simulink model "observer"  (R2021a)
settings: Solver=VariableStepAuto  StartTime=0.0  StopTime=0.25  MaxStep=0.0001  RelTol=1e-3
values from neighbouring files (symbols this model uses):
  A = adj    [ceren_function.m]    (also in deneme.m = [-resi/L -1/L; 1/C 0]; get_mass_spring_model.m = [0 1 0 0; (-k1-k2)/m1 0 k2/m1 0; 0 0 0 1; k2/m2 0 -k2/m2 0]; matlab.mat = [0  -100; 1000  0])
  B = [1/L; 0]    [deneme.m]    (also in get_mass_spring_model.m = [0; 1/m1; 0; 0]; matlab.mat = [100 0])
  c = 200    [init_graph.m]    (also in matlab.mat = 10)
  C = [0 1]    [deneme.m]    (also in get_mass_spring_model.m = [1 0 0 0; 0 0 1 0]; matlab.mat)
  c_switch = 1    [matlab.mat]
  D = [0]    [deneme.m]    (also in get_mass_spring_model.m = [0; 0; 0;0]; matlab.mat = 0)
  F = F'    [init_graph.m]    (also in matlab.mat = [-0.0499875062461 -10.4868971814])
  K = [7.50549770549 2.31662479036]    [matlab.mat]
settings Model: Creator=umut  LastModifiedBy=umut

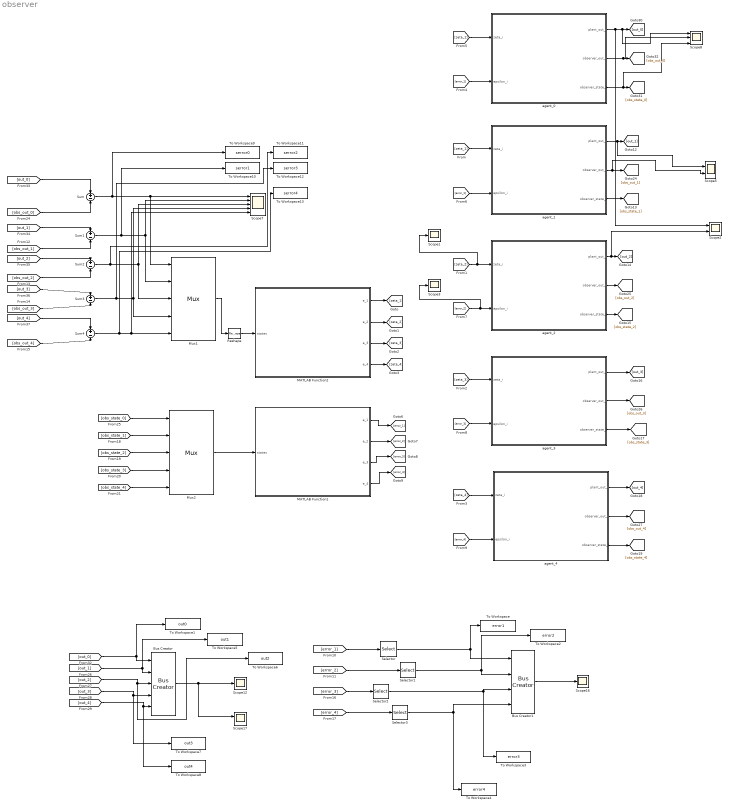
== system observer ==
  Bus Creator : BusCreator  Inputs=5
  Bus Creator1 : BusCreator  Inputs=4
  MATLAB Function1 : MATLAB Function  TreatAsAtomicUnit=on
  MATLAB Function2 : MATLAB Function  TreatAsAtomicUnit=on
  Mux1 : Mux  Inputs=5
  Mux2 : Mux  Inputs=5
  Reshape : Reshape  OutputDimensionality=Customize  OutputDimensions=[5,1]
  Scope{1,3,12,16} (4 alike) : Scope
  Scope17 : Scope  NumInputPorts=2
  Scope2 : Scope  NumInputPorts=2
  Scope5 : Scope  NumInputPorts=2
  Scope7 : Scope  NumInputPorts=5
  Scope8 : Scope  NumInputPorts=6
  Selector{,1..3} (4 alike) : Selector  InputPortWidth=2  IndexOptions=Starting index (dialog)  Indices=2  OutputSizes=1
  Sum{,1..4} (5 alike) : Sum  Inputs=+|-
  To Workspace : ToWorkspace  VariableName=error1  SampleTime=-1
      settings: Save2DSignal=2-D array (concatenate along first dimension)
  To Workspace1 : ToWorkspace  VariableName=out0  SampleTime=-1
      settings: Save2DSignal=2-D array (concatenate along first dimension)
  To Workspace10 : ToWorkspace  VariableName=serror1  SampleTime=-1
      settings: Save2DSignal=2-D array (concatenate along first dimension)
  To Workspace11 : ToWorkspace  VariableName=serror2  SampleTime=-1
      settings: Save2DSignal=2-D array (concatenate along first dimension)
  To Workspace12 : ToWorkspace  VariableName=serror3  SampleTime=-1
      settings: Save2DSignal=2-D array (concatenate along first dimension)
  To Workspace13 : ToWorkspace  VariableName=serror4  SampleTime=-1
      settings: Save2DSignal=2-D array (concatenate along first dimension)
  To Workspace2 : ToWorkspace  VariableName=error2  SampleTime=-1
      settings: Save2DSignal=2-D array (concatenate along first dimension)
  To Workspace3 : ToWorkspace  VariableName=error3  SampleTime=-1
      settings: Save2DSignal=2-D array (concatenate along first dimension)
  To Workspace4 : ToWorkspace  VariableName=error4  SampleTime=-1
      settings: Save2DSignal=2-D array (concatenate along first dimension)
  To Workspace5 : ToWorkspace  VariableName=out1  SampleTime=-1
      settings: Save2DSignal=2-D array (concatenate along first dimension)
  To Workspace6 : ToWorkspace  VariableName=out2  SampleTime=-1
      settings: Save2DSignal=2-D array (concatenate along first dimension)
  To Workspace7 : ToWorkspace  VariableName=out3  SampleTime=-1
      settings: Save2DSignal=2-D array (concatenate along first dimension)
  To Workspace8 : ToWorkspace  VariableName=out4  SampleTime=-1
      settings: Save2DSignal=2-D array (concatenate along first dimension)
  To Workspace9 : ToWorkspace  VariableName=serror0  SampleTime=-1
      settings: Save2DSignal=2-D array (concatenate along first dimension)
  agent_0 : Subsystem
  agent_1 : Subsystem
  agent_2 : Subsystem
  agent_3 : Subsystem
  agent_4 : Subsystem
  wires:
  MATLAB Function1/3(e_3) -> [error_3]
  MATLAB Function1/2(e_2) -> [error_2]
  MATLAB Function1/1(e_1) -> [error_1]
  MATLAB Function1/4(e_4) -> [error_4]
  [zeta_3] -> agent_3/1(zeta_i)
  [zeta_2] -> Scope1/1, agent_2/1(zeta_i)
  [zeta_4] -> agent_4/1(zeta_i)
  [error_3] -> agent_3/2(epsilon_i)
  [error_4] -> agent_4/2(epsilon_i)
  [error_2] -> Scope3/1, agent_2/2(epsilon_i)
  agent_1/3(observer_state_i) -> [obs_state_1]
  agent_2/1(plant_out_i) -> Scope2/2, [out_2]
  agent_2/3(observer_state_i) -> [obs_state_2]
  agent_3/1(plant_out_i) -> [out_3]
  agent_3/3(observer_state_i) -> [obs_state_3]
  agent_4/1(plant_out_i) -> [out_4]
  agent_4/3(observer_state_i) -> [obs_state_4]
  Mux1/1 -> Reshape/1
  Sum1/1 -> To Workspace10/1, Mux1/2, Scope7/2
  Sum2/1 -> To Workspace11/1, Scope7/3, Mux1/3
  Sum3/1 -> To Workspace12/1, Scope7/4, Mux1/4
  Sum4/1 -> To Workspace13/1, Scope7/5, Mux1/5
  agent_1/2(observer_out_i) -> Scope5/2, [obs_out_1]
  agent_2/2(observer_out_i) -> [obs_out_2]
  agent_3/2(observer_out_i) -> [obs_out_3]
  agent_4/2(observer_out_i) -> [obs_out_4]
  [obs_state_4] -> Mux2/5
  [obs_state_2] -> Mux2/3
  [obs_state_3] -> Mux2/4
  [obs_state_1] -> Mux2/2
  Mux2/1 -> MATLAB Function1/1(states)
  [error_1] -> agent_1/2(epsilon_i)
  [zeta_1] -> agent_1/1(zeta_i)
  agent_0/2(observer_out_i) -> Scope8/3, [obs_out_0]
  agent_0/3(observer_state_i) -> Scope8/6, [obs_state_0]
  Sum/1 -> To Workspace9/1, Mux1/1, Scope7/1
  [obs_state_0] -> Mux2/1
  [zeta_1] -> agent_0/1(zeta_i)
  [error_1] -> agent_0/2(epsilon_i)
  agent_0/1(plant_out_i) -> Scope2/1, Scope8/1, [out_0]
  [obs_out_0] -> Sum/2
  [out_0] -> Sum/1
  [obs_out_1] -> Sum1/2
  [out_1] -> Sum1/1
  [obs_out_2] -> Sum2/2
  [out_2] -> Sum2/1
  [obs_out_3] -> Sum3/2
  [out_3] -> Sum3/1
  [out_4] -> Sum4/1
  [obs_out_4] -> Sum4/2
  Reshape/1 -> MATLAB Function2/1(states)
  agent_1/1(plant_out_i) -> Scope5/1, [out_1]
  MATLAB Function2/3(e_3) -> [zeta_3]
  MATLAB Function2/4(e_4) -> [zeta_4]
  MATLAB Function2/2(e_2) -> [zeta_2]
  MATLAB Function2/1(e_1) -> [zeta_1]
  [out_3] -> To Workspace7/1, Bus Creator/4
  [out_4] -> To Workspace8/1, Bus Creator/5
  [out_2] -> To Workspace6/1, Bus Creator/3
  Bus Creator/1 -> Scope12/1, Scope17/1
  [out_0] -> Bus Creator/1, To Workspace1/1
  [out_1] -> Bus Creator/2, To Workspace5/1
  Selector/1 -> Bus Creator1/1, To Workspace/1
  Bus Creator1/1 -> Scope16/1
  Selector1/1 -> Bus Creator1/2, To Workspace2/1
  [error_1] -> Selector/1
  [error_2] -> Selector1/1
  [error_3] -> Selector2/1
  [error_4] -> Selector3/1
  Selector2/1 -> Bus Creator1/3, To Workspace3/1
  Selector3/1 -> To Workspace4/1, Bus Creator1/4

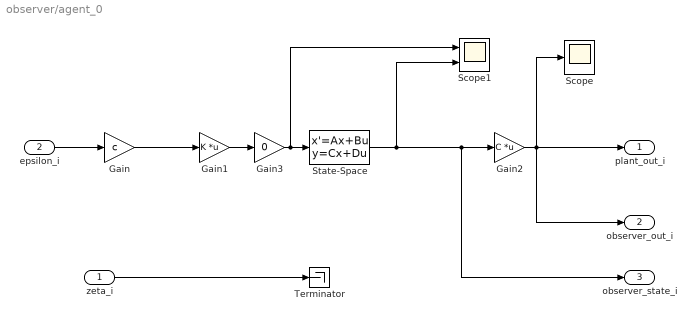
== system observer/agent_0 ==
  zeta_i : Inport
  epsilon_i : Inport  Port=2
  Gain : Gain  Gain=c
  Gain1 : Gain  Gain=K  Multiplication=Matrix(K*u)
  Gain2 : Gain  Gain=C  Multiplication=Matrix(K*u)
  Gain3 : Gain  Gain=0
  Scope : Scope
  Scope1 : Scope  NumInputPorts=2
  State-Space : StateSpace  A=A  B=B  C=eye(2)  D=[D;D]  InitialCondition=[20;0]
  Terminator : Terminator
  plant_out_i : Outport
  observer_out_i : Outport  Port=2
  observer_state_i : Outport  Port=3
  wires:
  epsilon_i/1 -> Gain/1
  zeta_i/1 -> Terminator/1
  State-Space/1 -> Scope1/2, Gain2/1, observer_state_i/1
  Gain/1 -> Gain1/1
  Gain2/1 -> Scope/1, plant_out_i/1, observer_out_i/1
  Gain1/1 -> Gain3/1
  Gain3/1 -> Scope1/1, State-Space/1

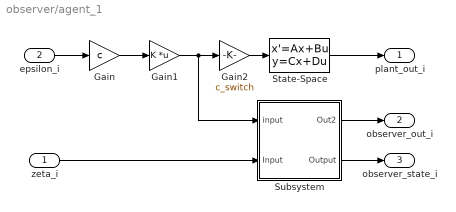
== system observer/agent_1 ==
  zeta_i : Inport
  epsilon_i : Inport  Port=2
  Gain : Gain  Gain=c
  Gain1 : Gain  Gain=K  Multiplication=Matrix(K*u)
  Gain2 : Gain  Gain=c_switch
  State-Space : StateSpace  A=A  B=B  C=C  D=D  InitialCondition=[30;80]
  Subsystem : Subsystem
  plant_out_i : Outport
  observer_out_i : Outport  Port=2
  observer_state_i : Outport  Port=3
  wires:
  epsilon_i/1 -> Gain/1
  State-Space/1 -> plant_out_i/1
  Subsystem/1(Out2) -> observer_out_i/1
  Subsystem/2(Output) -> observer_state_i/1
  zeta_i/1 -> Subsystem/2(Input)
  Gain/1 -> Gain1/1
  Gain1/1 -> Gain2/1, Subsystem/1(input)
  Gain2/1 -> State-Space/1

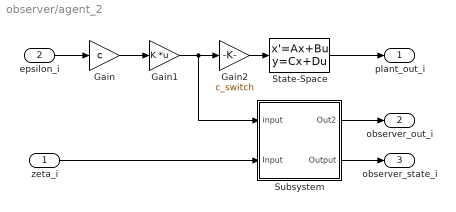
== system observer/agent_2 ==
  zeta_i : Inport
  epsilon_i : Inport  Port=2
  Gain : Gain  Gain=c
  Gain1 : Gain  Gain=K  Multiplication=Matrix(K*u)
  Gain2 : Gain  Gain=c_switch
  State-Space : StateSpace  A=A  B=B  C=C  D=D  InitialCondition=[30;100]
  Subsystem : Subsystem
  plant_out_i : Outport
  observer_out_i : Outport  Port=2
  observer_state_i : Outport  Port=3
  wires:
  epsilon_i/1 -> Gain/1
  State-Space/1 -> plant_out_i/1
  Subsystem/1(Out2) -> observer_out_i/1
  Subsystem/2(Output) -> observer_state_i/1
  zeta_i/1 -> Subsystem/2(Input)
  Gain/1 -> Gain1/1
  Gain1/1 -> Gain2/1, Subsystem/1(input)
  Gain2/1 -> State-Space/1

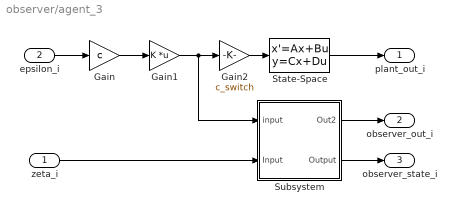
== system observer/agent_3 ==
  zeta_i : Inport
  epsilon_i : Inport  Port=2
  Gain : Gain  Gain=c
  Gain1 : Gain  Gain=K  Multiplication=Matrix(K*u)
  Gain2 : Gain  Gain=c_switch
  State-Space : StateSpace  A=A  B=B  C=C  D=D  InitialCondition=[20;60]
  Subsystem : Subsystem
  plant_out_i : Outport
  observer_out_i : Outport  Port=2
  observer_state_i : Outport  Port=3
  wires:
  epsilon_i/1 -> Gain/1
  State-Space/1 -> plant_out_i/1
  Subsystem/1(Out2) -> observer_out_i/1
  Subsystem/2(Output) -> observer_state_i/1
  zeta_i/1 -> Subsystem/2(Input)
  Gain/1 -> Gain1/1
  Gain1/1 -> Gain2/1, Subsystem/1(input)
  Gain2/1 -> State-Space/1

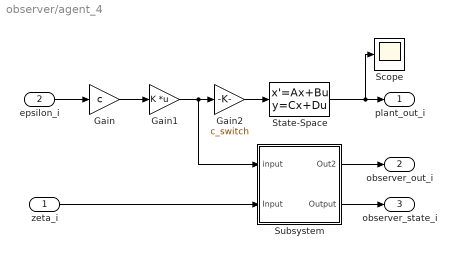
== system observer/agent_4 ==
  zeta_i : Inport
  epsilon_i : Inport  Port=2
  Gain : Gain  Gain=c
  Gain1 : Gain  Gain=K  Multiplication=Matrix(K*u)
  Gain2 : Gain  Gain=c_switch
  Scope : Scope
  State-Space : StateSpace  A=A  B=B  C=C  D=D  InitialCondition=[20;40]
  Subsystem : Subsystem
  plant_out_i : Outport
  observer_out_i : Outport  Port=2
  observer_state_i : Outport  Port=3
  wires:
  epsilon_i/1 -> Gain/1
  State-Space/1 -> Scope/1, plant_out_i/1
  Subsystem/1(Out2) -> observer_out_i/1
  Subsystem/2(Output) -> observer_state_i/1
  zeta_i/1 -> Subsystem/2(Input)
  Gain/1 -> Gain1/1
  Gain1/1 -> Gain2/1, Subsystem/1(input)
  Gain2/1 -> State-Space/1

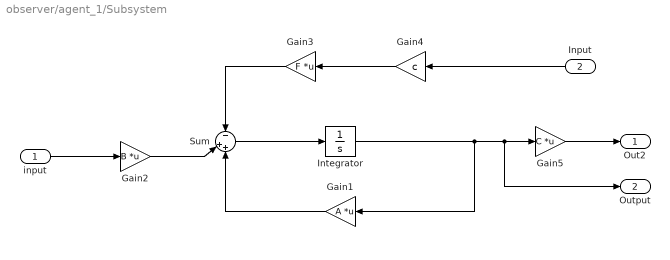
== system observer/agent_1/Subsystem ==
  input : Inport
  Input : Inport  Port=2
  Gain1 : Gain  Gain=A  Multiplication=Matrix(K*u)
  Gain2 : Gain  Gain=B  Multiplication=Matrix(K*u)
  Gain3 : Gain  Gain=F  Multiplication=Matrix(K*u)
  Gain4 : Gain  Gain=c
  Gain5 : Gain  Gain=C  Multiplication=Matrix(K*u)
  Integrator : Integrator
  Sum : Sum  Inputs=-|++
  Out2 : Outport
  Output : Outport  Port=2
  wires:
  Gain3/1 -> Sum/1
  Gain2/1 -> Sum/2
  input/1 -> Gain2/1
  Gain1/1 -> Sum/3
  Sum/1 -> Integrator/1
  Gain5/1 -> Out2/1
  Input/1 -> Gain4/1
  Gain4/1 -> Gain3/1
  Integrator/1 -> Output/1, Gain5/1, Gain1/1

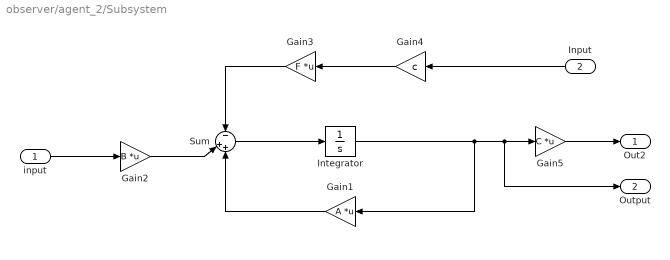
== system observer/agent_2/Subsystem ==
  input : Inport
  Input : Inport  Port=2
  Gain1 : Gain  Gain=A  Multiplication=Matrix(K*u)
  Gain2 : Gain  Gain=B  Multiplication=Matrix(K*u)
  Gain3 : Gain  Gain=F  Multiplication=Matrix(K*u)
  Gain4 : Gain  Gain=c
  Gain5 : Gain  Gain=C  Multiplication=Matrix(K*u)
  Integrator : Integrator
  Sum : Sum  Inputs=-|++
  Out2 : Outport
  Output : Outport  Port=2
  wires:
  Gain3/1 -> Sum/1
  Gain2/1 -> Sum/2
  input/1 -> Gain2/1
  Gain1/1 -> Sum/3
  Sum/1 -> Integrator/1
  Gain5/1 -> Out2/1
  Input/1 -> Gain4/1
  Gain4/1 -> Gain3/1
  Integrator/1 -> Output/1, Gain5/1, Gain1/1

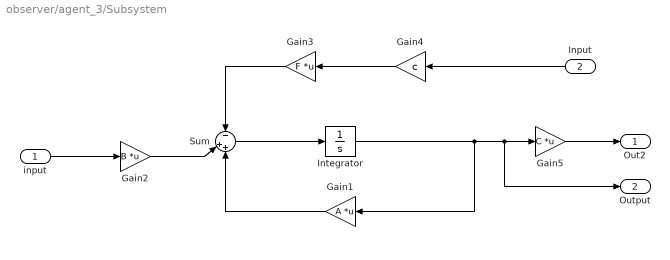
== system observer/agent_3/Subsystem ==
  input : Inport
  Input : Inport  Port=2
  Gain1 : Gain  Gain=A  Multiplication=Matrix(K*u)
  Gain2 : Gain  Gain=B  Multiplication=Matrix(K*u)
  Gain3 : Gain  Gain=F  Multiplication=Matrix(K*u)
  Gain4 : Gain  Gain=c
  Gain5 : Gain  Gain=C  Multiplication=Matrix(K*u)
  Integrator : Integrator
  Sum : Sum  Inputs=-|++
  Out2 : Outport
  Output : Outport  Port=2
  wires:
  Gain3/1 -> Sum/1
  Gain2/1 -> Sum/2
  input/1 -> Gain2/1
  Gain1/1 -> Sum/3
  Sum/1 -> Integrator/1
  Gain5/1 -> Out2/1
  Input/1 -> Gain4/1
  Gain4/1 -> Gain3/1
  Integrator/1 -> Output/1, Gain5/1, Gain1/1

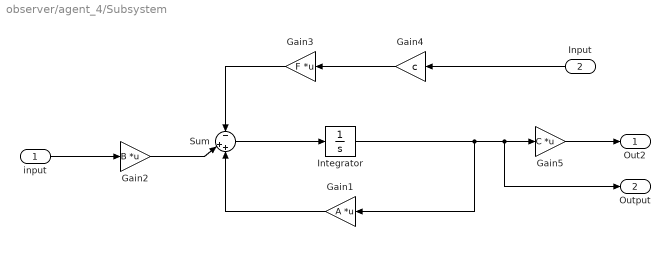
== system observer/agent_4/Subsystem ==
  input : Inport
  Input : Inport  Port=2
  Gain1 : Gain  Gain=A  Multiplication=Matrix(K*u)
  Gain2 : Gain  Gain=B  Multiplication=Matrix(K*u)
  Gain3 : Gain  Gain=F  Multiplication=Matrix(K*u)
  Gain4 : Gain  Gain=c
  Gain5 : Gain  Gain=C  Multiplication=Matrix(K*u)
  Integrator : Integrator
  Sum : Sum  Inputs=-|++
  Out2 : Outport
  Output : Outport  Port=2
  wires:
  Gain3/1 -> Sum/1
  Gain2/1 -> Sum/2
  input/1 -> Gain2/1
  Gain1/1 -> Sum/3
  Sum/1 -> Integrator/1
  Gain5/1 -> Out2/1
  Input/1 -> Gain4/1
  Gain4/1 -> Gain3/1
  Integrator/1 -> Output/1, Gain5/1, Gain1/1

== matlab function observer/MATLAB Function1 ==
  data: states input; e_1 output size=[2 1]; e_2 output size=[2 1]; e_3 output size=[2 1]; e_4 output size=[2 1]
function [e_1, e_2, e_3, e_4]  = calculate_neighborhood_error(states)
    adj = [ 0	1	1	1
            0   0   1   0
            1   0   0   0
            1   1   1   0]';
    
    pinnings = [1; 0; 0; 0];

    A = adj;
    G = pinnings;
    
    size_agents = 4;
    size_states = 2;
    
    error = zeros(size_states, size_agents);
    
    
    for i = 1 : size_agents
        error_temp = [0;0];
        for j = 1 : size_agents
            error_temp = error_temp + A(i, j) * (states((j)*2+1 : 2*(j+1)) - states((i)*2+1 : 2*(i+1)));
        end
        error_temp = error_temp + pinnings(i) * (states(1 : 2) - states((i)*2+1 : 2*(i+1)));
        error(:,i) = error_temp;
    end
    
    e_1 = error(:,1);
    e_2 = error(:,2);
    e_3 = error(:,3);
    e_4 = error(:,4);

end

== matlab function observer/MATLAB Function2 ==
  data: states input size=[5,1]; e_1 output size=[1, 1]; e_2 output size=[1, 1]; e_3 output size=[1, 1]; e_4 output size=[1, 1]
function [e_1, e_2, e_3, e_4]  = calculate_output_error(states)
    adj = [ 0	0	0	0
            1   0   0   0
            0   1   0   0
            0   0   1   0];
    
    pinnings = [1; 0; 0; 0];

    A = adj;
    G = pinnings;
    
    size_agents = 4;
    size_states = 1;
    
    error = zeros(size_states, size_agents);
    
    
    
    for i = 1 : size_agents
        error_temp = zeros(1,1);
        for j = 1 : size_agents
            term1 = (states(j+1) - states(i+1));
            error_temp = error_temp + A(i, j) * term1;
        end
        term2 = (states(1) - states(i+1 : (i+1)));
        error_temp = error_temp + pinnings(i) * term2;
        error(:,i) = error_temp;
    end
    
    e_1 = error(:,1);
    e_2 = error(:,2);
    e_3 = error(:,3);
    e_4 = error(:,4);

end
